simulink model "SENSOR_MODEL"  (R2019b)
settings: Solver=FixedStepDiscrete  StartTime=1  StopTime=11  FixedStep=1  RelTol=1e-3
settings Model: Creator=Bharti  LastModifiedBy=Bharti
settings ConfigComp: CovEnable=on  RecordCoverage=on  CovMetricSettings=dcmwe  CovModelRefEnable=on  DVTestSuiteOptimization=Auto  DVDetectOutOfBounds=on

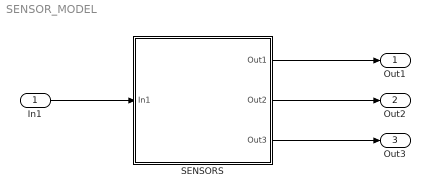
== system SENSOR_MODEL ==
  In1 : Inport
  SENSORS : Subsystem  TreatAsAtomicUnit=on
  Out1 : Outport
  Out2 : Outport  Port=2
  Out3 : Outport  Port=3
  wires:
  SENSORS/2(Out2) -> Out2/1
  SENSORS/1(Out1) -> Out1/1
  SENSORS/3(Out3) -> Out3/1
  In1/1 -> SENSORS/1(In1)

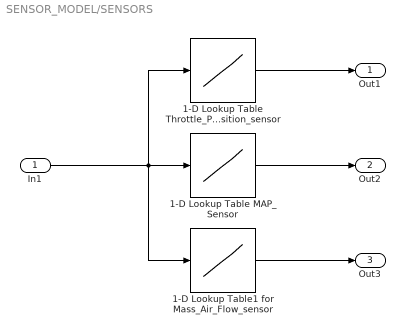
== system SENSOR_MODEL/SENSORS ==
  In1 : Inport
  1-D Lookup Table MAP_Sensor : Lookup_n-D  NumberOfTableDimensions=1  BreakpointsForDimension1=[800 3200]  Table=[0.3 1]  InternalRulePriority=Speed  RndMeth=Simplest  InputSameDT=on
  1-D Lookup Table Throttle_Position_sensor : Lookup_n-D  NumberOfTableDimensions=1  BreakpointsForDimension1=[800:240:3200]  Table=[0:10:100]  InternalRulePriority=Speed  RndMeth=Simplest  InputSameDT=on
  1-D Lookup Table1 for Mass_Air_Flow_sensor : Lookup_n-D  NumberOfTableDimensions=1  BreakpointsForDimension1=[800 3200]  Table=[7 25]  InternalRulePriority=Speed  RndMeth=Simplest  InputSameDT=on
  Out1 : Outport
  Out2 : Outport  Port=2
  Out3 : Outport  Port=3
  wires:
  In1/1 -> 1-D Lookup Table Throttle_Position_sensor/1, 1-D Lookup Table1 for Mass_Air_Flow_sensor/1, 1-D Lookup Table MAP_Sensor/1
  1-D Lookup Table1 for Mass_Air_Flow_sensor/1 -> Out3/1
  1-D Lookup Table MAP_Sensor/1 -> Out2/1
  1-D Lookup Table Throttle_Position_sensor/1 -> Out1/1
